simulink model "FOC_Motor_Control"  (R2020b)
settings: Solver=FixedStepDiscrete  StartTime=0.0  StopTime=10.0  FixedStep=Fixed_Step_Size  RelTol=1e-3
values from neighbouring files (symbols this model uses):
  Angle = 1.0    [Hall_HFI_FOC_Data.sldd]
  Cosine_table = 1.0 0.99999529 0.99999058 0.99998587 0.99998116 0.99996704 0.99995291 0.99993885 0.99992472 0.99990118 0.99987763 0.99985409 0.9998306 0.99979764 0.99976468 0.99973178 0.99969882 0.99965644 0.99961412 0.99957174 0.99952942 0.99947762 0.99942589 0.99937415 0.99932235 0.9992612 0.99920005 0.99913889 0.99907768 0.99900717 0.99893659 0.99886602 0.99879545 0.99871546 0.99863547 0.99855554 0.99847555 0.    [Hall_HFI_FOC_Data.sldd]
  Flux = 0.0027    [G474_FOC_HF.sldd]    (also in Hall_HFI_FOC_Data.sldd = 0.00529276
  HaLL_AngleShift = -0.25    [Hall_HFI_FOC_Data.sldd]
  HaLL_Sector1 = 5.236    [Hall_HFI_FOC_Data.sldd]
  HaLL_Sector2 = 1.0472    [Hall_HFI_FOC_Data.sldd]
  HaLL_Sector3 = 0.0    [Hall_HFI_FOC_Data.sldd]
  HaLL_Sector4 = 3.1415    [Hall_HFI_FOC_Data.sldd]
  HaLL_Sector5 = 4.1888    [Hall_HFI_FOC_Data.sldd]
  HaLL_Sector6 = 2.0944    [Hall_HFI_FOC_Data.sldd]
  HaLL_Timer_T = 1.0E-5    [Hall_HFI_FOC_Data.sldd]
  HFI_bw_BPF = 100.0    [Hall_HFI_FOC_Data.sldd]
  HFI_Fuc_Enalbe = 1.0    [Hall_HFI_FOC_Data.sldd]
  HFI_Inj_HF = 1000.0    [Hall_HFI_FOC_Data.sldd]
  HFI_Inj_HV = 2.0    [Hall_HFI_FOC_Data.sldd]
  HFI_IPD_F = 1000.0    [Hall_HFI_FOC_Data.sldd]
  HFI_IPD_Time = 0.1    [Hall_HFI_FOC_Data.sldd]
  HFI_IPD_V = 1.0    [Hall_HFI_FOC_Data.sldd]
  HFI_NS2RUN_Time = 0.1    [Hall_HFI_FOC_Data.sldd]
  HFI_NS_Low_Time = 0.01    [Hall_HFI_FOC_Data.sldd]
  HFI_NS_Time = 0.05    [Hall_HFI_FOC_Data.sldd]
  HFI_NS_V = 1.0    [Hall_HFI_FOC_Data.sldd]
  HFI_PI_Omega = 250.0    [Hall_HFI_FOC_Data.sldd]
  HFI_Pulse_Time = 0.001    [Hall_HFI_FOC_Data.sldd]
  HFI_Switch_Time = 0.1    [Hall_HFI_FOC_Data.sldd]
  ID_Ki = 45.0    [Hall_HFI_FOC_Data.sldd]
  ID_Kp = 0.4    [Hall_HFI_FOC_Data.sldd]
  inverter = struct    [PMSM_Parameters.m]
  IQ_Ki = 45.0    [Hall_HFI_FOC_Data.sldd]
  IQ_Kp = 0.45    [Hall_HFI_FOC_Data.sldd]
  LADRC_b0 = 80000.0    [Hall_HFI_FOC_Data.sldd]
  LADRC_Omega_c = 80.0    [Hall_HFI_FOC_Data.sldd]
  Ld = 4.9E-5    [G474_FOC_HF.sldd]    (also in Hall_HFI_FOC_Data.sldd = 0.0004
  Lq = 4.9E-5    [G474_FOC_HF.sldd]    (also in Hall_HFI_FOC_Data.sldd = 0.00045
  Over_modulation = 0.0    [Hall_HFI_FOC_Data.sldd]
  Pole_Pairs = 2.0    [Hall_HFI_FOC_Data.sldd]
  PWM_Frequency = 10000.0    [Hall_HFI_FOC_Data.sldd]
  R = 0.405    [Hall_HFI_FOC_Data.sldd]
  Sine_table = 0.0 0.0015339879 0.0030679768 0.0046019657 0.0061359555 0.0076698866 0.0092038177 0.010737749 0.012271681 0.013805497 0.015339312 0.016873131 0.018406944 0.019940587 0.021474229 0.023007872 0.024541514 0.026074925 0.027608337 0.029141748 0.03067516 0.032208283 0.033741407 0.035274528 0.036807653 0.038340431 0.039873205 0.04140598 0.042938754 0.04447113 0.046003502 0.047535874 0.049068246 0.0506001    [Hall_HFI_FOC_Data.sldd]
  SMO_K = 0.2    [Hall_HFI_FOC_Data.sldd]
  SMO_M = 0.1    [Hall_HFI_FOC_Data.sldd]
  SMO_PLL_W = 50.0    [Hall_HFI_FOC_Data.sldd]
  SMO_Theta_Enable = 0.0    [Hall_HFI_FOC_Data.sldd]
  Speed_Ki = 0.0633    [Hall_HFI_FOC_Data.sldd]
  Speed_Kp = 0.00867    [Hall_HFI_FOC_Data.sldd]
  Speed_PI_OutputMax = 6.0    [Hall_HFI_FOC_Data.sldd]
  Speed_PI_OutputMin = -6.0    [Hall_HFI_FOC_Data.sldd]
  SpeedFilter_Fn = 0.3    [Hall_HFI_FOC_Data.sldd]
  TorqueMode = 0.0    [Hall_HFI_FOC_Data.sldd]
undefined symbols (not defined in the file or in its folder): DiscIntNeverNeededParam, magnitude, SVPWM
libraries: simulink x6, eeGeneralControl x3, dspstat3 x3, pid_lib x2
(part 4 of 5)

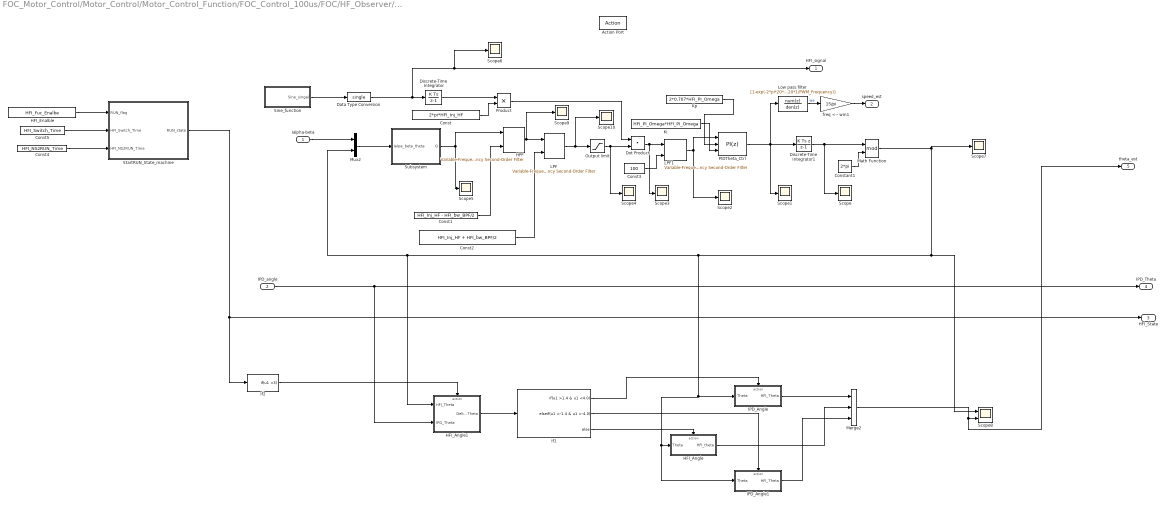
== system FOC_Motor_Control/Motor_Control/Motor_Control_Function/FOC_Control_100us/FOC/HF_Observer/HFI_Function/HFI ==
  Ialpha-beta : Inport
  IPD_angle : Inport  Port=2
  Action Port : ActionPort  ActionPortLabel=case [ 3 ]:
  Const : Constant  Value=2*pi*HFI_Inj_HF  OutDataTypeStr=single
  Const1 : Constant  Value=HFI_Inj_HF - HFI_bw_BPF/2  OutDataTypeStr=single
  Const2 : Constant  Value=HFI_Inj_HF + HFI_bw_BPF/2  OutDataTypeStr=single
  Const3 : Constant  Value=100  OutDataTypeStr=single
  Const4 : Constant  Value=HFI_NS2RUN_Time  OutDataTypeStr=single
  Const5 : Constant  Value=HFI_Switch_Time  OutDataTypeStr=single
  Constant1 : Constant  Value=2*pi  OutDataTypeStr=single
  Data Type Conversion : DataTypeConversion  OutDataTypeStr=single
  Discrete-Time Integrator : DiscreteIntegrator  SampleTime=-1  ICPrevOutput=DiscIntNeverNeededParam  ICPrevScaledInput=DiscIntNeverNeededParam
  Discrete-Time Integrator1 : DiscreteIntegrator  IntegratorMethod=Integration: Backward Euler  SampleTime=-1  ICPrevOutput=DiscIntNeverNeededParam  ICPrevScaledInput=DiscIntNeverNeededParam
  Dot Product : DotProduct  InputSameDT=on  OutDataTypeStr=Inherit: Inherit via internal rule
  HFI_Angle : Subsystem
  HFI_Angle1 : Subsystem
  HFI_Enalble : Constant  Value=HFI_Fuc_Enalbe  VectorParams1D=off  OutDataTypeStr=uint8
  HPF : eeGeneralControl/Variable-Frequency Second-Order Filter  FilterType=High-pass  fn=60  Zeta=single(0.3)  Ts=-1  A0=0  Ph0=0  f0=0  b0=0
      settings: SourceProductBaseCode=PS
  IPD_Angle : Subsystem
  IPD_Angle1 : Subsystem
  If1 : If  IfExpression=u1 >1.4 & u1 <4.0  ElseIfExpressions=u1 <-1.4 & u1 >-4.0
  If2 : If  IfExpression=u1 <3  ShowElse=off
  Ki : Constant  Value=HFI_PI_Omega*HFI_PI_Omega  OutDataTypeStr=single
  Kp : Constant  Value=2*0.707*HFI_PI_Omega  OutDataTypeStr=single
  LPF : eeGeneralControl/Variable-Frequency Second-Order Filter  FilterType=Low-pass  fn=60  Zeta=single(0.3)  Ts=-1  A0=0  Ph0=0  f0=0  b0=0
      settings: SourceProductBaseCode=PS
  LPF1 : eeGeneralControl/Variable-Frequency Second-Order Filter  FilterType=Low-pass  fn=60  Zeta=single(0.707)  Ts=-1  A0=0  Ph0=0  f0=0  b0=0
      settings: SourceProductBaseCode=PS
  Low pass filter : DiscreteTransferFcn  Numerator=[1-exp(-2*pi*20*1/PWM_Frequency)]  Denominator=[1 -exp(-2*pi*20*1/PWM_Frequency)]
  Math Function : Math  Operator=mod  SignedPower=on  SaturateOnIntegerOverflow=on
  Merge2 : Merge  Inputs=3
  Mux2 : Mux  Inputs=2
  Output limit : Saturate
  PIDTheta_Ctrl : pid_lib/PID Controller  Controller=PI  Form=Parallel  TimeDomain=Discrete-time  UseExternalTs=off  SampleTime=-1  IntegratorMethod=Forward Euler  FilterMethod=Forward Euler  ControllerParametersSource=external  P=2*0.707*SMO_PLL_W  I=SMO_PLL_W*SMO_PLL_W  D=0  UseFilter=on  N=100  TunerSelectOption=Transfer Function Based (PID Tuner App)  ZeroCross=off  InitialConditionSource=internal  InitialConditionForIntegrator=1  InitialConditionForFilter=0  DifferentiatorICPrevScaledInput=0  ExternalReset=none  TrackingMode=off  Kt=1  LimitOutput=on  SatLimitsSource=internal  UpperSaturationLimit=2*pi*500  LowerSaturationLimit=-2*pi*500  LinearizeAsGain=off  AntiWindupMode=clamping  Kb=50  POutMin=[]  POutMax=[]  IOutMin=[]  IOutMax=[]  DOutMin=[]  DOutMax=[]  NOutMin=[]  NOutMax=[]  SumOutMin=[]  SumOutMax=[]  SaturationOutDataTypeStr=Inherit: Inherit via back propagation  SaturationOutMin=[]  SaturationOutMax=[]  PParamMin=[]  PParamMax=[]  IParamMin=[]  IParamMax=[]  DParamMin=[]  DParamMax=[]  NParamMin=[]  NParamMax=[]  KbParamMin=[]  KbParamMax=[]  KtParamMin=[]  KtParamMax=[]  KbOutMin=[]  KbOutMax=[]  KtOutMin=[]  KtOutMax=[]  IntegratorOutMin=[]  IntegratorOutMax=[]  FilterOutMin=[]  FilterOutMax=[]  SumI1OutMin=[]  SumI1OutMax=[]  SumI2OutMin=[]  SumI2OutMax=[]  SumI3OutMin=[]  SumI3OutMax=[]  SumI4OutMin=[]  SumI4OutMax=[]  SumDOutMin=[]  SumDOutMax=[]  DifferentiatorOutMin=[]  DifferentiatorOutMax=[]  FilterDiffOutCoefMin=[]  FilterDiffOutCoefMax=[]  ReciprocalOutMin=[]  ReciprocalOutMax=[]  SumDenOutMin=[]  SumDenOutMax=[]  SumNumOutMin=[]  SumNumOutMax=[]  DivideOutMin=[]  DivideOutMax=[]  UdiffTsProdOutMin=[]  UdiffTsProdOutMax=[]  NTsProdOutMin=[]  NTsProdOutMax=[]  UintegralTsProdOutMin=[]  UintegralTsProdOutMax=[]  UngainTsProdOutMin=[]  UngainTsProdOutMax=[]  IntegratorContinuousStateAttributes=''  IntegratorStateMustResolveToSignalObject=off  IntegratorRTWStateStorageClass=Auto  FilterContinuousStateAttributes=''  FilterStateMustResolveToSignalObject=off  FilterRTWStateStorageClass=Auto  ParallelPVariant=ExternalParameters  IdealPVariant=Disabled  IVariant=ExternalParameters  DVariant=Disabled  IntegratorVariant=Discrete  SatVariant=Enabled  AWVariant=DiscClampingParallel  PCopyVariant=Disabled  TRVariant=Disabled  FdbkBlocksVariant=Forward  IdealPFdbkVariant=Disabled  SatFdbkVariant=Disabled  DerivativeFilterVariant=Disabled  NVariant=Disabled  NCopyVariant=Disabled_SignalSpec  FilterICVariant=Disabled  IntegratorICVariant=InternalICs  ExternalResetVariant=Disabled  TRSumVariant=Passthrough  SumFdbkVariant=Disabled  SumVariant=Sum_PI  TsampFilterVariant=InternalTs  TsampNgainVariant=Passthrough  TsampIntegralVariant=Passthrough  ExternalSaturationOutDataTypeStr=Inherit: Same as second input
  Product : Product
  Scope{,1..7,9..10} (10 alike) : Scope
  Scope8 : Scope  NumInputPorts=2
  Sine_function : Subsystem
      settings: RTWSystemCode=Nonreusable function  RTWFcnNameOpts=Use subsystem name
  StartRUN_State_machine : Stateflow chart  TreatAsAtomicUnit=on
      settings: RTWSystemCode=Nonreusable function  RTWFcnNameOpts=Use subsystem name
  Subsystem : Subsystem
  freq <-- wm1 : Gain  Gain=15/pi
  HFI_signal : Outport
  speed_est : Outport  Port=2
  HFI_State : Outport  Port=3
  IPD_Theta : Outport  Port=4
  theta_est : Outport  Port=5
  wires:
  Mux2/1 -> Subsystem/1(Ialpa_beta_theta)
  Ialpha-beta/1 -> Mux2/1
  Subsystem/1(Q) -> Scope5/1, HPF/1
  freq <-- wm1/1 -> speed_est/1
  Discrete-Time Integrator1/1 -> Scope/1, Math Function/1
  LPF1/1 -> PIDTheta_Ctrl/1, Scope2/1
  Low pass filter/1 -> freq <-- wm1/1  "we"
  Discrete-Time Integrator/1 -> Product/1
  Product/1 -> Dot Product/1
  Dot Product/1 -> Scope3/1, LPF1/1
  Constant1/1 -> Math Function/2
  LPF/1 -> Output limit/1, Scope10/1
  Const/1 -> Product/2
  Sine_function/1(Sine_singal) -> Data Type Conversion/1
  Data Type Conversion/1 -> Scope6/1, HFI_signal/1, Discrete-Time Integrator/1
  HFI_Enalble/1 -> StartRUN_State_machine/1(RUN_flag)
  StartRUN_State_machine/1(RUN_state) -> If2/1, HFI_State/1
  IPD_angle/1 -> HFI_Angle1/2(IPD_Theta), IPD_Theta/1
  Math Function/1 -> IPD_Angle1/1(Theta), HFI_Angle/1(Theta), IPD_Angle/1(Theta), HFI_Angle1/1(HFI_Theta), Mux2/2, Scope8/1, Scope7/1
  PIDTheta_Ctrl/1 -> Scope1/1, Low pass filter/1, Discrete-Time Integrator1/1
  If1/1 -> IPD_Angle/Action
  HFI_Angle/1(HFI_theta) -> Merge2/2
  If1/3 -> HFI_Angle/Action
  IPD_Angle/1(HFI_Theta) -> Merge2/1
  HFI_Angle1/1(Delta_Theta) -> If1/1
  If2/1 -> HFI_Angle1/Action
  Merge2/1 -> theta_est/1, Scope8/2
  If1/2 -> IPD_Angle1/Action
  IPD_Angle1/1(HFI_Theta) -> Merge2/3
  Const1/1 -> HPF/2
  Const2/1 -> LPF/2
  Const3/1 -> LPF1/2
  Const5/1 -> StartRUN_State_machine/2(HFI_Switch_Time)
  Const4/1 -> StartRUN_State_machine/3(HFI_NS2RUN_Time)
  HPF/1 -> Scope9/1, LPF/1
  Ki/1 -> PIDTheta_Ctrl/3
  Kp/1 -> PIDTheta_Ctrl/2
  Output limit/1 -> Scope4/1, Dot Product/2

== system FOC_Motor_Control/Motor_Control/Motor_Control_Function/FOC_Control_100us/FOC/HF_Observer/HFI_Function/IPD ==
  Iabc : Inport  PortDimensions=3
  Action Port : ActionPort  ActionPortLabel=case [ 1 ]:
  7 : Fcn  Expr=u[1]*u[3]
  8 : Fcn  Expr=u[1]*u[2]
  Constant : Constant  Value=HFI_IPD_V
  Demux1 : Demux  Outputs=3
  HF_Angle : Subsystem
  Mux : Mux  Inputs=3
  Scope : Scope
  Sine_Cosine : Subsystem  TreatAsAtomicUnit=on
      settings: RTWSystemCode=Nonreusable function  RTWFcnNameOpts=Use subsystem name
  Theta_cacl : Subsystem
      settings: RTWSystemCode=Nonreusable function
  Ualpha : Outport
  Ubeta : Outport  Port=2
  Theta : Outport  Port=3
  wires:
  Sine_Cosine/1(Sin) -> Mux/2
  Sine_Cosine/2(Cos) -> Mux/3
  Constant/1 -> Mux/1
  Mux/1 -> 8/1, 7/1
  7/1 -> Ualpha/1
  8/1 -> Ubeta/1
  Iabc/1 -> Scope/1, Demux1/1  "Phase_CurrentABC"
  HF_Angle/1(Theta_V) -> Sine_Cosine/1(P)
  Demux1/3 -> Theta_cacl/3(Ic)
  Demux1/2 -> Theta_cacl/2(Ib)
  Theta_cacl/1(Theta) -> Theta/1
  Demux1/1 -> Theta_cacl/1(Ia)

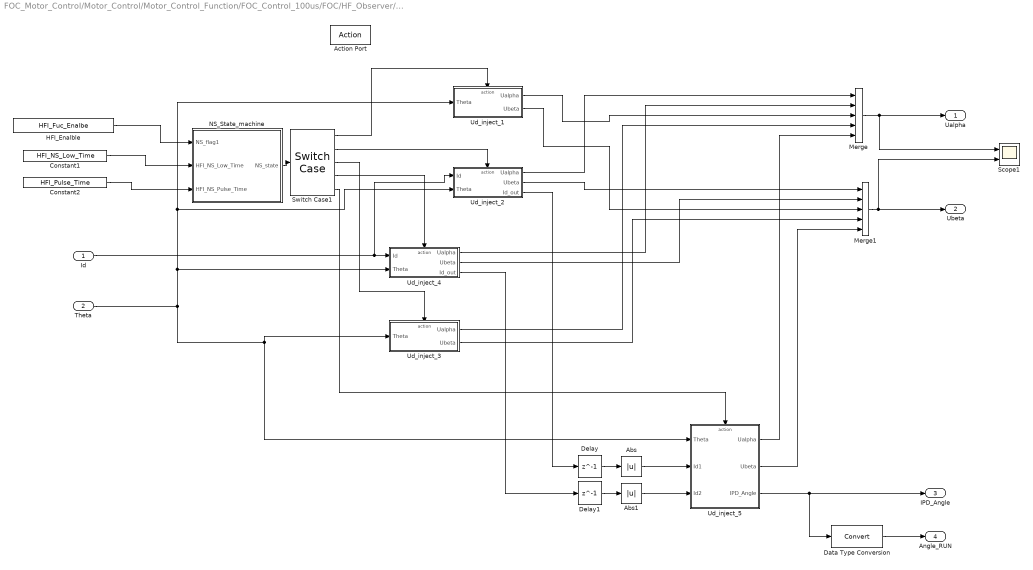
== system FOC_Motor_Control/Motor_Control/Motor_Control_Function/FOC_Control_100us/FOC/HF_Observer/HFI_Function/NS ==
  Id : Inport
  Theta : Inport  Port=2
  Action Port : ActionPort  ActionPortLabel=case [ 2 ]:
  Abs : Abs
  Abs1 : Abs
  Constant1 : Constant  Value=HFI_NS_Low_Time  OutDataTypeStr=single
  Constant2 : Constant  Value=HFI_Pulse_Time  OutDataTypeStr=single
  Data Type Conversion : DataTypeConversion
  Delay : Delay  DelayLength=1  InitialCondition=0
  Delay1 : Delay  DelayLength=1  InitialCondition=0
  HFI_Enalble : Constant  Value=HFI_Fuc_Enalbe  OutDataTypeStr=uint8
  Merge : Merge  Inputs=5
  Merge1 : Merge  Inputs=5
  NS_State_machine : Stateflow chart  TreatAsAtomicUnit=on
      settings: RTWSystemCode=Nonreusable function  RTWFcnNameOpts=Use subsystem name
  Scope1 : Scope  NumInputPorts=2
  Switch Case1 : SwitchCase  CaseConditions={1,2,3,4,5}  ShowDefaultCase=off
  Ud_inject_1 : Subsystem
  Ud_inject_2 : Subsystem
  Ud_inject_3 : Subsystem
  Ud_inject_4 : Subsystem
  Ud_inject_5 : Subsystem
  Ualpha : Outport
  Ubeta : Outport  Port=2
  IPD_Angle : Outport  Port=3
  Angle_RUN : Outport  Port=4
  wires:
  HFI_Enalble/1 -> NS_State_machine/1(NS_flag1)
  NS_State_machine/1(NS_state) -> Switch Case1/1
  Id/1 -> Ud_inject_2/1(Id), Ud_inject_4/1(Id)
  Merge/1 -> Scope1/1, Ualpha/1
  Ud_inject_2/1(Ualpha) -> Merge/1
  Ud_inject_4/1(Ualpha) -> Merge/2
  Merge1/1 -> Scope1/2, Ubeta/1
  Ud_inject_2/2(Ubeta) -> Merge1/1
  Ud_inject_4/2(Ubeta) -> Merge1/2
  Ud_inject_4/3(Id_out) -> Delay1/1
  Ud_inject_2/3(Id_out) -> Delay/1
  Ud_inject_1/1(Ualpha) -> Merge/3
  Ud_inject_1/2(Ubeta) -> Merge1/3
  Ud_inject_3/1(Ualpha) -> Merge/4
  Ud_inject_3/2(Ubeta) -> Merge1/4
  Switch Case1/1 -> Ud_inject_1/Action
  Switch Case1/2 -> Ud_inject_2/Action
  Theta/1 -> Ud_inject_4/2(Theta), Ud_inject_2/2(Theta), Ud_inject_1/1(Theta), Ud_inject_5/1(Theta), Ud_inject_3/1(Theta)
  Switch Case1/3 -> Ud_inject_3/Action
  Switch Case1/4 -> Ud_inject_4/Action
  Switch Case1/5 -> Ud_inject_5/Action
  Ud_inject_5/1(Ualpha) -> Merge/5
  Ud_inject_5/2(Ubeta) -> Merge1/5
  Abs/1 -> Ud_inject_5/2(Id1)
  Abs1/1 -> Ud_inject_5/3(Id2)
  Ud_inject_5/3(IPD_Angle) -> Data Type Conversion/1, IPD_Angle/1
  Delay/1 -> Abs/1
  Delay1/1 -> Abs1/1
  Data Type Conversion/1 -> Angle_RUN/1
  Constant1/1 -> NS_State_machine/2(HFI_NS_Low_Time)
  Constant2/1 -> NS_State_machine/3(HFI_NS_Pulse_Time)

== system FOC_Motor_Control/Motor_Control/Motor_Control_Function/FOC_Control_100us/FOC/HIGH_SMO/QPLL/Sine_Cosine ==
  note: Sine Cosine Coefficients
  P : Inport
  Cosine : Lookup_n-D  NumberOfTableDimensions=1  LookupTableObject=''  BreakpointsForDimension1=[0:2*pi/4095:2*pi]  BreakpointsForDimension1FirstPoint=10  BreakpointsForDimension2FirstPoint=10  BreakpointsForDimension1Spacing=12  BreakpointsForDimension2Spacing=12  IndexSearchMethod=Evenly spaced points  Table=Cosine_table  InterpMethod=Flat  DiagnosticForOutOfRangeInput=Error  InternalRulePriority=Speed  RndMeth=Simplest  InputSameDT=on
  Saturation : Saturate  UpperLimit=2*pi-0.0001  LowerLimit=0+0.0001
  Scope : Scope  NumInputPorts=2
  Sine : Lookup_n-D  NumberOfTableDimensions=1  LookupTableObject=''  BreakpointsForDimension1=[0:2*pi/4095:2*pi]  BreakpointsForDimension1FirstPoint=10  BreakpointsForDimension2FirstPoint=10  BreakpointsForDimension1Spacing=12  BreakpointsForDimension2Spacing=12  IndexSearchMethod=Evenly spaced points  Table=Sine_table  InterpMethod=Flat  DiagnosticForOutOfRangeInput=Error  InternalRulePriority=Speed  RndMeth=Simplest  InputSameDT=on
  Cos : Outport  VectorParamsAs1DForOutWhenUnconnected=off
  Sin : Outport  Port=2  VectorParamsAs1DForOutWhenUnconnected=off
  wires:
  P/1 -> Saturation/1  "position"
  Sine/1 -> Scope/1, Sin/1
  Cosine/1 -> Scope/2, Cos/1
  Saturation/1 -> Cosine/1, Sine/1

== system FOC_Motor_Control/Motor_Control/Motor_Control_Function/FOC_Control_100us/FOC/HIGH_SMO/QPLL/SpeedToTheta ==
  In1 : Inport
  RangeLimit : Subsystem
  Sum1 : Sum  Inputs=|++
  Ts : Gain  Gain=1/PWM_Frequency
  Unit Delay : UnitDelay  SampleTime=-1  HasFrameUpgradeWarning=on
  Out1 : Outport
  wires:
  In1/1 -> Ts/1
  Ts/1 -> Sum1/1
  Sum1/1 -> RangeLimit/1(In)
  Unit Delay/1 -> Out1/1, Sum1/2
  RangeLimit/1(Theta) -> Unit Delay/1

== system FOC_Motor_Control/Motor_Control/Motor_Control_Function/FOC_Control_100us/FOC/HIGH_SMO/QPLL/Subsystem1 ==
  Err_in : Inport
  speed : Inport  Port=2
  If : If
  If Action Subsystem : Subsystem  TreatAsAtomicUnit=on
  If Action Subsystem1 : Subsystem  TreatAsAtomicUnit=on
  Merge : Merge
  Product : Product
  Out : Outport  VectorParamsAs1DForOutWhenUnconnected=off
  wires:
  speed/1 -> If/1
  Merge/1 -> Product/1
  Err_in/1 -> Product/2
  Product/1 -> Out/1
  If/1 -> If Action Subsystem/Action
  If Action Subsystem/1(Out1) -> Merge/1
  If Action Subsystem1/1(Out1) -> Merge/2
  If/2 -> If Action Subsystem1/Action

== system FOC_Motor_Control/Motor_Control/Motor_Control_Function/FOC_Control_100us/FOC/Q_Current_PI/IQ_Control/Normal ==
  Bus_voltage : Inport
  Action Port : ActionPort  ActionPortLabel=elseif(u1==0)
  Gain : Gain  Gain=1/sqrt(3)
  Gain1 : Gain  Gain=-1/sqrt(3)
  Out1 : Outport
  Out2 : Outport  Port=2
  wires:
  Bus_voltage/1 -> Gain1/1, Gain/1
  Gain/1 -> Out1/1
  Gain1/1 -> Out2/1

== system FOC_Motor_Control/Motor_Control/Motor_Control_Function/FOC_Control_100us/FOC/Q_Current_PI/IQ_Control/Over_M ==
  Bus_voltage : Inport
  Action Port : ActionPort  ActionPortLabel=if(u1==1)
  Gain : Gain  Gain=2/3
  Gain1 : Gain  Gain=-2/3
  Out1 : Outport
  Out2 : Outport  Port=2
  wires:
  Bus_voltage/1 -> Gain1/1, Gain/1
  Gain/1 -> Out1/1
  Gain1/1 -> Out2/1

== system FOC_Motor_Control/Motor_Control/Motor_Control_Function/Control_Command_2ms/Control_Command_2ms/Speed_PI/Speed_PI/Speed_Control/Speed_Control ==
  Err : Inport
  Action Port : ActionPort  ActionPortLabel=if((u1==3)&(u2==1))
  Add : Sum
  Cons : Constant  Value=0  OutDataTypeStr=single
  Discrete-Time Integrator : DiscreteIntegrator  SampleTime=-1  ICPrevOutput=DiscIntNeverNeededParam  ICPrevScaledInput=DiscIntNeverNeededParam
  Ki : Constant  Value=Speed_Ki  OutDataTypeStr=single
  Kp : Constant  Value=Speed_Kp  OutDataTypeStr=single
  Product : Product
  Product1 : Product
  Relational Operator1 : RelationalOperator  Operator===  OutDataTypeStr=boolean  RndMeth=Simplest
  Saturation : Saturate  UpperLimit=Speed_PI_OutputMax  LowerLimit=Speed_PI_OutputMin
  Scope : Scope
  Switch : Switch  Criteria=u2 > Threshold
  Unit Delay3 : UnitDelay  SampleTime=-1  HasFrameUpgradeWarning=on
  PI_Out : Outport
  wires:
  Kp/1 -> Product/1
  Err/1 -> Switch/1, Product/2
  Switch/1 -> Product1/2
  Product1/1 -> Discrete-Time Integrator/1
  Product/1 -> Add/1
  Add/1 -> Relational Operator1/1, Saturation/1
  Saturation/1 -> Relational Operator1/2, PI_Out/1
  Discrete-Time Integrator/1 -> Add/2, Scope/1
  Relational Operator1/1 -> Unit Delay3/1
  Ki/1 -> Product1/1
  Unit Delay3/1 -> Switch/2
  Cons/1 -> Switch/3

== system FOC_Motor_Control/Motor_Control/Motor_Control_Function/Control_Command_2ms/Control_Command_2ms/Speed_PI/Speed_PI/Speed_Control/Speed_Control1 ==
  Err : Inport
  Action Port : ActionPort  ActionPortLabel=elseif((u2==0))
  Add : Sum
  Cons : Constant  Value=0  OutDataTypeStr=single
  Discrete-Time Integrator : DiscreteIntegrator  SampleTime=-1  ICPrevOutput=DiscIntNeverNeededParam  ICPrevScaledInput=DiscIntNeverNeededParam
  Ki : Constant  Value=Speed_Ki  OutDataTypeStr=single
  Kp : Constant  Value=Speed_Kp  OutDataTypeStr=single
  Product : Product
  Product1 : Product
  Relational Operator1 : RelationalOperator  Operator===  OutDataTypeStr=boolean  RndMeth=Simplest
  Saturation : Saturate  UpperLimit=Speed_PI_OutputMax  LowerLimit=Speed_PI_OutputMin
  Switch : Switch  Criteria=u2 > Threshold
  Unit Delay3 : UnitDelay  SampleTime=-1  HasFrameUpgradeWarning=on
  PI_Out : Outport
  wires:
  Kp/1 -> Product/1
  Err/1 -> Switch/1, Product/2
  Switch/1 -> Product1/2
  Product1/1 -> Discrete-Time Integrator/1
  Product/1 -> Add/1
  Add/1 -> Saturation/1, Relational Operator1/1
  Saturation/1 -> Relational Operator1/2, PI_Out/1
  Discrete-Time Integrator/1 -> Add/2
  Relational Operator1/1 -> Unit Delay3/1
  Ki/1 -> Product1/1
  Unit Delay3/1 -> Switch/2
  Cons/1 -> Switch/3

== system FOC_Motor_Control/Motor_Control/Motor_Control_Function/FOC_Control_100us/FOC/HF_Observer/HFI_Function/HFI/HFI_Angle ==
  Theta : Inport
  Action Port : ActionPort  ActionPortLabel=else
  HFI_theta : Outport
  wires:
  Theta/1 -> HFI_theta/1

== system FOC_Motor_Control/Motor_Control/Motor_Control_Function/FOC_Control_100us/FOC/HF_Observer/HFI_Function/HFI/HFI_Angle1 ==
  HFI_Theta : Inport
  IPD_Theta : Inport  Port=2
  Action Port : ActionPort  ActionPortLabel=if(u1 <3)
  Subtract : Sum  Inputs=+-
  Delta_Theta : Outport
  wires:
  HFI_Theta/1 -> Subtract/1
  IPD_Theta/1 -> Subtract/2
  Subtract/1 -> Delta_Theta/1

== system FOC_Motor_Control/Motor_Control/Motor_Control_Function/FOC_Control_100us/FOC/HF_Observer/HFI_Function/HFI/IPD_Angle ==
  Theta : Inport
  Action Port : ActionPort  ActionPortLabel=if(u1 >1.4 & u1 <4.0)
  Angle_calibration : Subsystem  TreatAsAtomicUnit=on
      settings: RTWSystemCode=Nonreusable function  RTWFcnNameOpts=Use subsystem name
  HFI_Theta : Outport
  wires:
  Theta/1 -> Angle_calibration/1(Angle_input)
  Angle_calibration/1(Angle_output) -> HFI_Theta/1

== system FOC_Motor_Control/Motor_Control/Motor_Control_Function/FOC_Control_100us/FOC/HF_Observer/HFI_Function/HFI/IPD_Angle1 ==
  Theta : Inport
  Action Port : ActionPort  ActionPortLabel=elseif(u1 <-1.4 & u1 >-4.0)
  Angle_calibration : Subsystem  TreatAsAtomicUnit=on
      settings: RTWSystemCode=Nonreusable function  RTWFcnNameOpts=Use subsystem name
  HFI_Theta : Outport
  wires:
  Theta/1 -> Angle_calibration/1(Angle_input)
  Angle_calibration/1(Angle_output) -> HFI_Theta/1

== system FOC_Motor_Control/Motor_Control/Motor_Control_Function/FOC_Control_100us/FOC/HF_Observer/HFI_Function/HFI/Sine_function ==
  A : Gain  Gain=HFI_Inj_HV
  Add : Sum
  Const1 : Constant  Value=2*pi*1*HFI_Inj_HF/PWM_Frequency  OutDataTypeStr=single
  Const2 : Constant  Value=2*pi  OutDataTypeStr=single
  Const3 : Constant  Value=0  OutDataTypeStr=single
  Const4 : Constant  OutDataTypeStr=single
  Delay : Delay  DelayLength=1  InitialCondition=0
  Memory : Memory  InheritSampleTime=on
  Product1 : Product
  Relational Operator1 : RelationalOperator  Operator=<  OutDataTypeStr=boolean  RndMeth=Simplest
  Sine : Lookup_n-D  NumberOfTableDimensions=1  LookupTableObject=''  BreakpointsForDimension1=[0:2*pi/4095:2*pi]  BreakpointsForDimension1FirstPoint=10  BreakpointsForDimension2FirstPoint=10  BreakpointsForDimension1Spacing=12  BreakpointsForDimension2Spacing=12  IndexSearchMethod=Evenly spaced points  Table=Sine_table  InterpMethod=Flat  DiagnosticForOutOfRangeInput=Error  InternalRulePriority=Speed  RndMeth=Simplest  InputSameDT=on
  Switch : Switch  Criteria=u2 > Threshold
  Sine_singal : Outport
  wires:
  Switch/1 -> Product1/1
  Const3/1 -> Switch/3
  Relational Operator1/1 -> Switch/2
  Delay/1 -> Relational Operator1/1
  Const2/1 -> Relational Operator1/2
  Add/1 -> Memory/1, Delay/1
  Sine/1 -> A/1
  Product1/1 -> Sine/1, Add/2
  Memory/1 -> Product1/2
  Const1/1 -> Add/1
  Const4/1 -> Switch/1
  A/1 -> Sine_singal/1

== system FOC_Motor_Control/Motor_Control/Motor_Control_Function/FOC_Control_100us/FOC/HF_Observer/HFI_Function/HFI/Subsystem ==
  Ialpa_beta_theta : Inport
  Add2 : Sum  Inputs=-+  OutDataTypeStr=Inherit: Same as first input
  Demux : Demux  Outputs=2
  Demux1 : Demux  Outputs=2
  Produc3t : Product  RndMeth=Simplest  OutDataTypeStr=Inherit: Same as first input
  Product4 : Product  RndMeth=Simplest  OutDataTypeStr=Inherit: Same as first input
  Sine_Cosine : Subsystem
      settings: RTWSystemCode=Nonreusable function  RTWFcnNameOpts=Use subsystem name
  Q : Outport  VectorParamsAs1DForOutWhenUnconnected=off
  wires:
  Add2/1 -> Q/1
  Sine_Cosine/2(Cos) -> Product4/2
  Produc3t/1 -> Add2/1
  Sine_Cosine/1(Sin) -> Produc3t/2
  Product4/1 -> Add2/2
  Demux/1 -> Produc3t/1
  Demux/2 -> Product4/1
  Demux1/1 -> Demux/1
  Demux1/2 -> Sine_Cosine/1(P)
  Ialpa_beta_theta/1 -> Demux1/1

== system FOC_Motor_Control/Motor_Control/Motor_Control_Function/FOC_Control_100us/FOC/HF_Observer/HFI_Function/IPD/HF_Angle ==
  Add : Sum
  Const1 : Constant  Value=2*pi*HFI_IPD_F/PWM_Frequency  OutDataTypeStr=single
  Const2 : Constant  Value=2*pi  OutDataTypeStr=single
  Const3 : Constant  Value=0  OutDataTypeStr=single
  Const4 : Constant  OutDataTypeStr=single
  Delay : Delay  DelayLength=1  InitialCondition=0
  Memory : Memory  InheritSampleTime=on
  Product1 : Product
  Relational Operator1 : RelationalOperator  Operator=<  OutDataTypeStr=boolean  RndMeth=Simplest
  Switch : Switch  Criteria=u2 > Threshold
  Theta_V : Outport
  wires:
  Switch/1 -> Product1/1
  Delay/1 -> Relational Operator1/1
  Const2/1 -> Relational Operator1/2
  Const3/1 -> Switch/3
  Relational Operator1/1 -> Switch/2
  Const1/1 -> Add/1
  Memory/1 -> Product1/2
  Add/1 -> Memory/1, Delay/1
  Product1/1 -> Theta_V/1, Add/2
  Const4/1 -> Switch/1

== system FOC_Motor_Control/Motor_Control/Motor_Control_Function/FOC_Control_100us/FOC/HF_Observer/HFI_Function/IPD/Sine_Cosine ==
  note: Sine Cosine Coefficients
  P : Inport
  Cosine : Lookup_n-D  NumberOfTableDimensions=1  LookupTableObject=''  BreakpointsForDimension1=[0:2*pi/4095:2*pi]  BreakpointsForDimension1FirstPoint=10  BreakpointsForDimension2FirstPoint=10  BreakpointsForDimension1Spacing=12  BreakpointsForDimension2Spacing=12  IndexSearchMethod=Evenly spaced points  Table=Cosine_table  InterpMethod=Flat  DiagnosticForOutOfRangeInput=Error  InternalRulePriority=Speed  RndMeth=Simplest  InputSameDT=on
  Scope : Scope  NumInputPorts=2
  Sine : Lookup_n-D  NumberOfTableDimensions=1  LookupTableObject=''  BreakpointsForDimension1=[0:2*pi/4095:2*pi]  BreakpointsForDimension1FirstPoint=10  BreakpointsForDimension2FirstPoint=10  BreakpointsForDimension1Spacing=12  BreakpointsForDimension2Spacing=12  IndexSearchMethod=Evenly spaced points  Table=Sine_table  InterpMethod=Flat  DiagnosticForOutOfRangeInput=Error  InternalRulePriority=Speed  RndMeth=Simplest  InputSameDT=on
  Sin : Outport  VectorParamsAs1DForOutWhenUnconnected=off
  Cos : Outport  Port=2  VectorParamsAs1DForOutWhenUnconnected=off
  wires:
  P/1 -> Cosine/1, Sine/1  "position"
  Sine/1 -> Scope/1, Sin/1
  Cosine/1 -> Scope/2, Cos/1

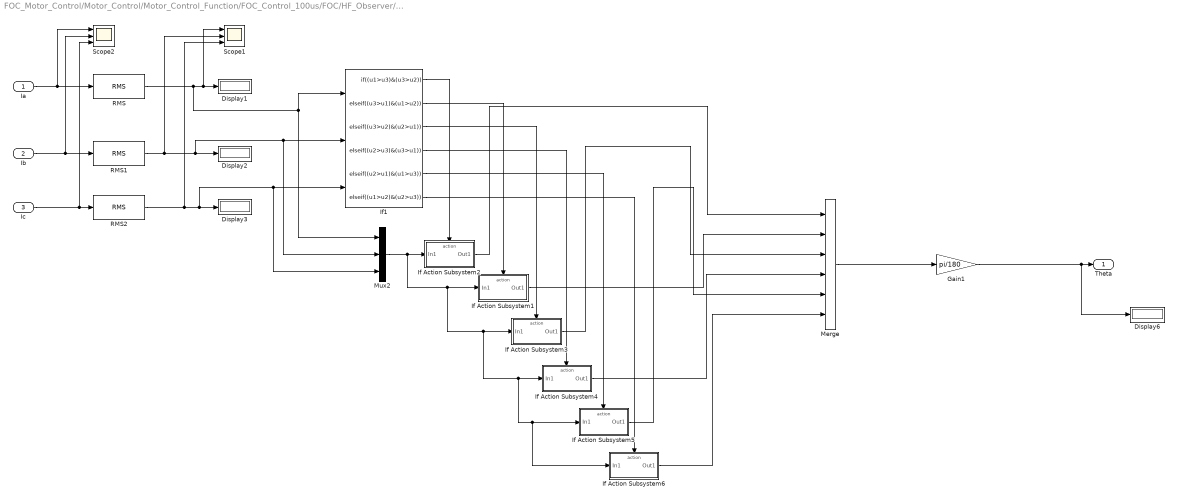
== system FOC_Motor_Control/Motor_Control/Motor_Control_Function/FOC_Control_100us/FOC/HF_Observer/HFI_Function/IPD/Theta_cacl ==
  Ia : Inport
  Ib : Inport  Port=2
  Ic : Inport  Port=3
  Display{1..3,6} (4 alike) : Display
  Gain1 : Gain  Gain=pi/180
  If Action Subsystem1 : Subsystem  TreatAsAtomicUnit=on
  If Action Subsystem2 : Subsystem  TreatAsAtomicUnit=on
  If Action Subsystem3 : Subsystem  TreatAsAtomicUnit=on
  If Action Subsystem4 : Subsystem  TreatAsAtomicUnit=on
  If Action Subsystem5 : Subsystem  TreatAsAtomicUnit=on
  If Action Subsystem6 : Subsystem  TreatAsAtomicUnit=on
  If1 : If  NumInputs=3  IfExpression=(u1>u3)&(u3>u2)  ElseIfExpressions=(u3>u1)&(u1>u2),(u3>u2)&(u2>u1),(u2>u3)&(u3>u1),(u2>u1)&(u1>u3),(u1>u2)&(u2>u3)  ShowElse=off
  Merge : Merge  Inputs=6
  Mux2 : Mux  Inputs=3
  RMS : dspstat3/RMS  run=on  directionMode=Each column  dimension=1  reset_popup=None
  RMS1 : dspstat3/RMS  run=on  directionMode=Each column  dimension=1  reset_popup=None
  RMS2 : dspstat3/RMS  run=on  directionMode=Each column  dimension=1  InputProcessing=Columns as channels (frame based)  reset_popup=None
  Scope1 : Scope  NumInputPorts=3
  Scope2 : Scope  NumInputPorts=3
  Theta : Outport
  wires:
  Ia/1 -> Scope2/1, RMS/1
  Ib/1 -> Scope2/2, RMS1/1
  Ic/1 -> Scope2/3, RMS2/1
  RMS2/1 -> Mux2/3, If1/3, Display3/1, Scope1/3
  RMS1/1 -> Mux2/2, If1/2, Display2/1, Scope1/2
  RMS/1 -> If1/1, Mux2/1, Display1/1, Scope1/1
  If1/1 -> If Action Subsystem2/Action
  If1/2 -> If Action Subsystem1/Action
  If1/3 -> If Action Subsystem3/Action
  If1/4 -> If Action Subsystem4/Action
  If1/5 -> If Action Subsystem5/Action
  If1/6 -> If Action Subsystem6/Action
  Mux2/1 -> If Action Subsystem6/1(In1), If Action Subsystem5/1(In1), If Action Subsystem4/1(In1), If Action Subsystem3/1(In1), If Action Subsystem1/1(In1), If Action Subsystem2/1(In1)
  If Action Subsystem2/1(Out1) -> Merge/1
  If Action Subsystem1/1(Out1) -> Merge/2
  If Action Subsystem3/1(Out1) -> Merge/3
  If Action Subsystem4/1(Out1) -> Merge/4
  If Action Subsystem5/1(Out1) -> Merge/5
  If Action Subsystem6/1(Out1) -> Merge/6
  Merge/1 -> Gain1/1
  Gain1/1 -> Display6/1, Theta/1

== system FOC_Motor_Control/Motor_Control/Motor_Control_Function/FOC_Control_100us/FOC/HF_Observer/HFI_Function/NS/Ud_inject_1 ==
  Theta : Inport
  Action Port : ActionPort  ActionPortLabel=case [ 1 ]:
  1 : Fcn  Expr=u[1]*u[4]-u[2]*u[3]
  2 : Fcn  Expr=u[1]*u[3]+u[2]*u[4]
  Constant : Constant  Value=0  OutDataTypeStr=single
  Constant2 : Constant  Value=0  OutDataTypeStr=single
  Mux : Mux
  Sine_Cosine : Subsystem  TreatAsAtomicUnit=on
      settings: RTWSystemCode=Nonreusable function  RTWFcnNameOpts=Use subsystem name
  Ualpha : Outport
  Ubeta : Outport  Port=2
  wires:
  Constant2/1 -> Mux/2
  Theta/1 -> Sine_Cosine/1(P)
  2/1 -> Ubeta/1
  Sine_Cosine/2(Cos) -> Mux/4
  1/1 -> Ualpha/1
  Constant/1 -> Mux/1
  Mux/1 -> 2/1, 1/1
  Sine_Cosine/1(Sin) -> Mux/3

== system FOC_Motor_Control/Motor_Control/Motor_Control_Function/FOC_Control_100us/FOC/HF_Observer/HFI_Function/NS/Ud_inject_2 ==
  Id : Inport
  Theta : Inport  Port=2
  Action Port : ActionPort  ActionPortLabel=case [ 2 ]:
  1 : Fcn  Expr=u[1]*u[4]-u[2]*u[3]
  2 : Fcn  Expr=u[1]*u[3]+u[2]*u[4]
  Constant : Constant  Value=HFI_NS_V  OutDataTypeStr=single
  Constant2 : Constant  Value=0  OutDataTypeStr=single
  Mux : Mux
  Sine_Cosine : Subsystem  TreatAsAtomicUnit=on
      settings: RTWSystemCode=Nonreusable function  RTWFcnNameOpts=Use subsystem name
  Ualpha : Outport
  Ubeta : Outport  Port=2
  Id_out : Outport  Port=3
  wires:
  Constant2/1 -> Mux/2
  Theta/1 -> Sine_Cosine/1(P)
  2/1 -> Ubeta/1
  Sine_Cosine/2(Cos) -> Mux/4
  1/1 -> Ualpha/1
  Constant/1 -> Mux/1
  Mux/1 -> 2/1, 1/1
  Sine_Cosine/1(Sin) -> Mux/3
  Id/1 -> Id_out/1

== system FOC_Motor_Control/Motor_Control/Motor_Control_Function/FOC_Control_100us/FOC/HF_Observer/HFI_Function/NS/Ud_inject_3 ==
  Theta : Inport
  Action Port : ActionPort  ActionPortLabel=case [ 3 ]:
  1 : Fcn  Expr=u[1]*u[4]-u[2]*u[3]
  2 : Fcn  Expr=u[1]*u[3]+u[2]*u[4]
  Constant : Constant  Value=0  OutDataTypeStr=single
  Constant2 : Constant  Value=0  OutDataTypeStr=single
  Mux : Mux
  Sine_Cosine : Subsystem  TreatAsAtomicUnit=on
      settings: RTWSystemCode=Nonreusable function  RTWFcnNameOpts=Use subsystem name
  Ualpha : Outport
  Ubeta : Outport  Port=2
  wires:
  Constant2/1 -> Mux/2
  Theta/1 -> Sine_Cosine/1(P)
  2/1 -> Ubeta/1
  Sine_Cosine/2(Cos) -> Mux/4
  1/1 -> Ualpha/1
  Constant/1 -> Mux/1
  Mux/1 -> 2/1, 1/1
  Sine_Cosine/1(Sin) -> Mux/3

== system FOC_Motor_Control/Motor_Control/Motor_Control_Function/FOC_Control_100us/FOC/HF_Observer/HFI_Function/NS/Ud_inject_4 ==
  Id : Inport
  Theta : Inport  Port=2
  Action Port : ActionPort  ActionPortLabel=case [ 4 ]:
  1 : Fcn  Expr=u[1]*u[4]-u[2]*u[3]
  2 : Fcn  Expr=u[1]*u[3]+u[2]*u[4]
  Constant : Constant  Value=HFI_NS_V  OutDataTypeStr=single
  Constant2 : Constant  Value=0  OutDataTypeStr=single
  Mux : Mux
  Sine_Cosine : Subsystem  TreatAsAtomicUnit=on
      settings: RTWSystemCode=Nonreusable function
  Theta_limit : Subsystem
      settings: RTWSystemCode=Nonreusable function
  Ualpha : Outport
  Ubeta : Outport  Port=2
  Id_out : Outport  Port=3
  wires:
  Constant2/1 -> Mux/2
  2/1 -> Ubeta/1
  Sine_Cosine/2(Cos) -> Mux/4
  1/1 -> Ualpha/1
  Constant/1 -> Mux/1
  Mux/1 -> 2/1, 1/1
  Sine_Cosine/1(Sin) -> Mux/3
  Id/1 -> Id_out/1
  Theta_limit/1(Angle_output) -> Sine_Cosine/1(P)
  Theta/1 -> Theta_limit/1(Angle_input)

== system FOC_Motor_Control/Motor_Control/Motor_Control_Function/FOC_Control_100us/FOC/HF_Observer/HFI_Function/NS/Ud_inject_5 ==
  Theta : Inport
  Id1 : Inport  Port=2
  Id2 : Inport  Port=3
  Action Port : ActionPort  ActionPortLabel=case [ 5 ]:
  1 : Fcn  Expr=u[1]*u[4]-u[2]*u[3]
  2 : Fcn  Expr=u[1]*u[3]+u[2]*u[4]
  Constant : Constant  Value=0  OutDataTypeStr=single
  Constant2 : Constant  Value=0  OutDataTypeStr=single
  If1 : If  NumInputs=2  IfExpression=u1>=u2  ElseIfExpressions=u1<u2  ShowElse=off
  Merge1 : Merge
  Mux : Mux
  Sine_Cosine : Subsystem
      settings: RTWSystemCode=Nonreusable function  RTWFcnNameOpts=Use subsystem name
  Subsystem : Subsystem
  Subsystem1 : Subsystem
  Ualpha : Outport
  Ubeta : Outport  Port=2
  IPD_Angle : Outport  Port=3
  wires:
  Constant2/1 -> Mux/2
  Theta/1 -> Subsystem1/1(In1), Subsystem/1(In1), Sine_Cosine/1(P)
  2/1 -> Ubeta/1
  Sine_Cosine/2(Cos) -> Mux/4
  1/1 -> Ualpha/1
  Constant/1 -> Mux/1
  Mux/1 -> 2/1, 1/1
  Sine_Cosine/1(Sin) -> Mux/3
  Id1/1 -> If1/1
  Id2/1 -> If1/2
  If1/1 -> Subsystem/Action
  If1/2 -> Subsystem1/Action
  Subsystem/1(Out1) -> Merge1/1
  Subsystem1/1(Out1) -> Merge1/2
  Merge1/1 -> IPD_Angle/1
